simulink model "FxLMS_Model"  (R2026a)
settings: Solver=FixedStepDiscrete  StopTime=15  FixedStep=1/8000
values from neighbouring files (symbols this model uses):
  mu_W = 0.05 * mu_max    [FxLMS_Simulation.m]
  true_secondary_path = [0, 0, 0.1, 0.8, 0.3, -0.2, 0.05]    [FxLMS_Simulation.m]
undefined symbols (not defined in the file or in its folder): dspblkCoreblockFVToolHelper, gcbh
libraries: simulink x1
settings Model: Creator=ojasv  LastModifiedBy=ojasv

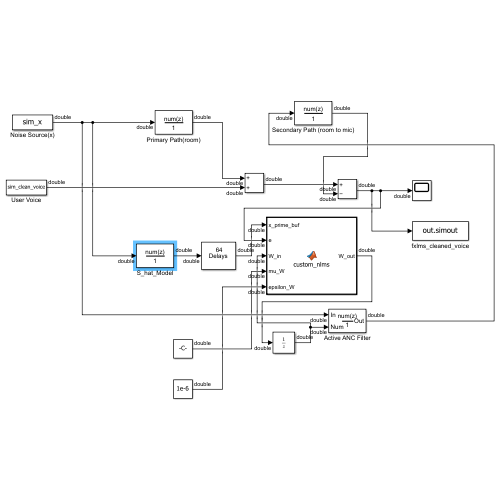
[thumbnail: Simulink's stored preview of the top-level diagram]
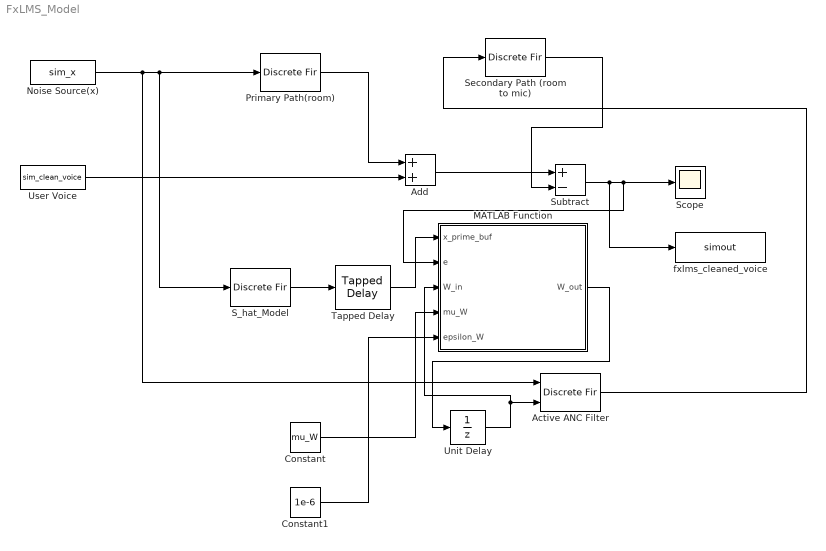
== system FxLMS_Model ==
  Active ANC Filter : DiscreteFir  LoadFcn=dspblkCoreblockFVToolHelper(gcbh,'load');  CoefSource=Input port
      settings: CopyFcn=dspblkCoreblockFVToolHelper(gcbh,'copy');  DeleteFcn=dspblkCoreblockFVToolHelper(gcbh,'close');  ModelCloseFcn=dspblkCoreblockFVToolHelper(gcbh,'close');  PreSaveFcn=dspblkCoreblockFVToolHelper(gcbh,'presave');  PostSaveFcn=dspblkCoreblockFVToolHelper(gcbh,'postsave');  CloseFcn=dspblkCoreblockFVToolHelper(gcbh,'close');  InputPortMap=u0,u1
  Add : Sum
  Constant : Constant  Value=mu_W
  Constant1 : Constant  Value=1e-6
  MATLAB Function : MATLAB Function  TreatAsAtomicUnit=on
  Noise Source(x) : FromWorkspace  VariableName=sim_x  SampleTime=1/8000
  Primary Path(room) : DiscreteFir  LoadFcn=dspblkCoreblockFVToolHelper(gcbh,'load');  Coefficients=room_path'
      settings: CopyFcn=dspblkCoreblockFVToolHelper(gcbh,'copy');  DeleteFcn=dspblkCoreblockFVToolHelper(gcbh,'close');  ModelCloseFcn=dspblkCoreblockFVToolHelper(gcbh,'close');  PreSaveFcn=dspblkCoreblockFVToolHelper(gcbh,'presave');  PostSaveFcn=dspblkCoreblockFVToolHelper(gcbh,'postsave');  CloseFcn=dspblkCoreblockFVToolHelper(gcbh,'close');
  S_hat_Model : DiscreteFir  LoadFcn=dspblkCoreblockFVToolHelper(gcbh,'load');  Coefficients=S_hat'
      settings: CopyFcn=dspblkCoreblockFVToolHelper(gcbh,'copy');  DeleteFcn=dspblkCoreblockFVToolHelper(gcbh,'close');  ModelCloseFcn=dspblkCoreblockFVToolHelper(gcbh,'close');  PreSaveFcn=dspblkCoreblockFVToolHelper(gcbh,'presave');  PostSaveFcn=dspblkCoreblockFVToolHelper(gcbh,'postsave');  CloseFcn=dspblkCoreblockFVToolHelper(gcbh,'close');
  Scope : Scope
      settings: ActiveDisplayYMinimum=-33.441445506836217  ActiveDisplayYMaximum=17.909182547737938
  Secondary Path (room to mic) : DiscreteFir  LoadFcn=dspblkCoreblockFVToolHelper(gcbh,'load');  Coefficients=true_secondary_path
      settings: CopyFcn=dspblkCoreblockFVToolHelper(gcbh,'copy');  DeleteFcn=dspblkCoreblockFVToolHelper(gcbh,'close');  ModelCloseFcn=dspblkCoreblockFVToolHelper(gcbh,'close');  PreSaveFcn=dspblkCoreblockFVToolHelper(gcbh,'presave');  PostSaveFcn=dspblkCoreblockFVToolHelper(gcbh,'postsave');  CloseFcn=dspblkCoreblockFVToolHelper(gcbh,'close');
  Subtract : Sum  Inputs=+-
  Tapped Delay : simulink/Discrete/Tapped Delay  vinit=0.0  samptime=-1  NumDelays=64  DelayOrder=Oldest  includeCurrent=off
  Unit Delay : UnitDelay  SampleTime=-1
  User Voice : FromWorkspace  VariableName=sim_clean_voice  SampleTime=1/8000
  fxlms_cleaned_voice : ToWorkspace  VariableName=simout  SampleTime=-1
  wires:
  Noise Source(x)/1 -> Active ANC Filter/1, S_hat_Model/1, Primary Path(room)/1
  User Voice/1 -> Add/2
  Primary Path(room)/1 -> Add/1
  Add/1 -> Subtract/1
  Secondary Path (room to mic)/1 -> Subtract/2
  Subtract/1 -> MATLAB Function/2(e), Scope/1, fxlms_cleaned_voice/1
  Active ANC Filter/1 -> Secondary Path (room to mic)/1
  S_hat_Model/1 -> Tapped Delay/1
  Tapped Delay/1 -> MATLAB Function/1(x_prime_buf)
  Constant/1 -> MATLAB Function/4(mu_W)
  Constant1/1 -> MATLAB Function/5(epsilon_W)
  Unit Delay/1 -> MATLAB Function/3(W_in), Active ANC Filter/2
  MATLAB Function/1(W_out) -> Unit Delay/1

== matlab function FxLMS_Model/MATLAB Function ==
  data: x_prime_buf input; W_out output; e input; W_in input; mu_W input; epsilon_W input
function W_out = custom_nlms(x_prime_buf, e, W_in, mu_W, epsilon_W)
% Calculate adaptive step size
mu_adaptive = mu_W / (epsilon_W + norm(x_prime_buf)^2);

% Use .* for strict element-wise multiplication against the buffer
W_out = W_in + (mu_adaptive * e) .* x_prime_buf;
end
